simulink model "BoatLibraryTest02"  (R2013b)
settings: Solver=ode45  StartTime=0.0  StopTime=10  RelTol=1e-3
values from neighbouring files (symbols this model uses):
  C = C0    [Minimizer.m]    (also in parameters2.m = [1 0 0 0 0 0;0 0 1 0 0 0;0 0 0 0 1 0]; parameters3.m = [1 0 0 0 0 0;0 0 1 0 0 0;0 0 0 0 1 0])
  fw = 4    [parameters2.m]    (also in parameters3.m)
  I = 1/12*M*((2*rx1)^2 + (2*ry1)^2)    (= 7.46230507536)    [BoatController.m]    (also in boatDynamics.m; parameters2.m = 20; parameters3.m)
  inputBound = [minInput maxInput]    [parameters3.m]
  kr = 2    [parameters2.m]    (also in parameters3.m)
  M = 80*lbtokg    (= 36.28736)    [BoatController.m]    (also in parameters2.m = 10; parameters3.m)
  rx1 = -12*intom    (= -0.3048)    [BoatController.m]    (also in boatDynamics.m; costfunction.m; parameters3.m)
  rx2 = 12*intom    (= 0.3048)    [BoatController.m]    (also in boatDynamics.m; costfunction.m; parameters3.m)
  ry1 = -69*intom/2 + 6*intom    (= -0.7239)    [BoatController.m]    (also in boatDynamics.m; costfunction.m; parameters3.m)
  ry2 = ry1    (= -0.7239)    [BoatController.m]    (also in boatDynamics.m; costfunction.m; parameters3.m)
undefined symbols (not defined in the file): K
libraries: simulink x6
settings Model: Creator=Darsan  LastModifiedBy=darsan13
settings DataIOCC: SignalLoggingSaveFormat=ModelDataLogs
settings OptimizationCC: ExpressionDepthLimit=2147483647
settings DebuggingCC: FcnCallInpInsideContextMsg=EnableAllAsWarning  StateNameClashWarn=warning

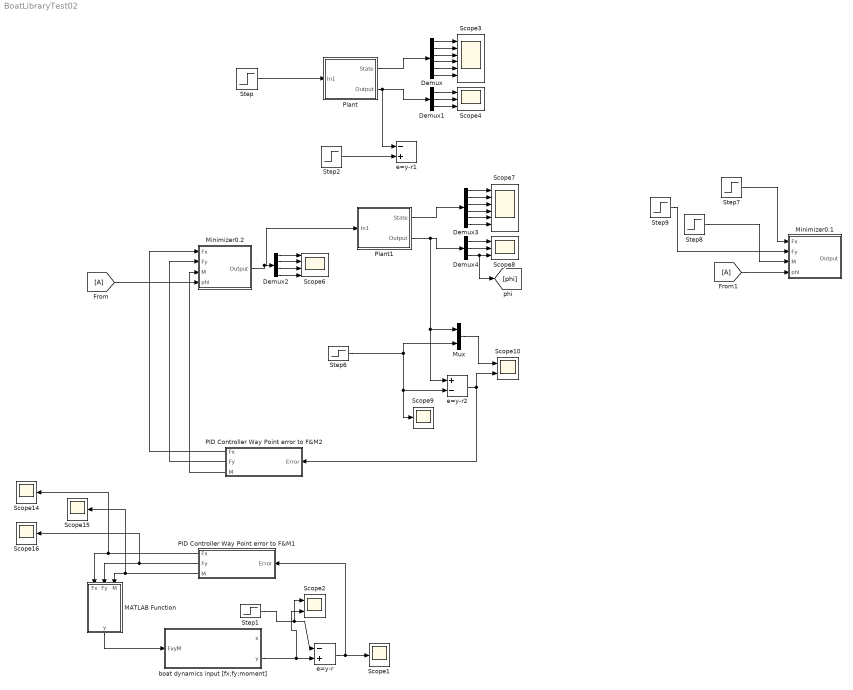
== system BoatLibraryTest02 ==
  Demux : Demux  Outputs=6
  Demux1 : Demux  Outputs=3
  Demux2 : Demux
  Demux3 : Demux  Outputs=6
  Demux4 : Demux  Outputs=3
  MATLAB Function : MATLAB Function  TreatAsAtomicUnit=on
  Minimizer0.1 : Subsystem  mask{rx1=rx1, rx2=rx2, ry1=ry1, ry2=ry2, C=K, inputBound=inputBound}
      mask prompts: C "Performance Gain"; inputBound "Input Bounds"
  Minimizer0.2 : Subsystem  mask{rx1=rx1, rx2=rx2, ry1=ry1, ry2=ry2, C=K, inputBound=inputBound}
      mask prompts: C "Performance Gain"; inputBound "Input Bounds"
  Mux : Mux  Inputs=2
  PID Controller Way Point error to F&M1 : Subsystem
  PID Controller Way Point error to F&M2 : Subsystem
  Plant : Subsystem  mask{rx1=rx1, rx2=rx2, ry1=ry1, ry2=ry2, M=M, I=I, C=C}
      mask TypeOptions rx1: Constant/Value
  Plant1 : Subsystem  mask{rx1=rx1, rx2=rx2, ry1=ry1, ry2=ry2, M=M, I=I, C=C}
      mask TypeOptions rx1: Constant/Value
  Scope{1,9,14..16} (5 alike) : Scope
      Scope1 settings: YMin=-3  YMax=0  SaveName=ScopeData2
      Scope14 settings: YMin=50  YMax=260  SaveName=ScopeData13
      Scope15 settings: YMin=50  YMax=260  SaveName=ScopeData14
      Scope16 settings: YMin=50  YMax=260  SaveName=ScopeData15
      Scope9 settings: SaveName=ScopeData8
  Scope10 : Scope  NumInputPorts=2
      settings: YMin=-22.5~-22.5  YMax=7.5~5  SaveName=ScopeData9
  Scope2 : Scope  NumInputPorts=2
      settings: YMin=-5~-5  YMax=5~5
  Scope3 : Scope  NumInputPorts=6
      settings: YMin=-250000~-4.5~-5~-5~-5~-5  YMax=250000~4.5~5~5~5~5
  Scope4 : Scope  NumInputPorts=3
      settings: YMin=-250000~-4.5~-5  YMax=250000~4.5~5  SaveName=ScopeData3
  Scope6 : Scope  NumInputPorts=4
      settings: YMin=100~100~50~55  YMax=100~100~50~100  SaveName=ScopeData5
  Scope7 : Scope  NumInputPorts=6
      settings: YMin=-250000~-4.5~-5~-5~-5~-5  YMax=250000~4.5~5~5~5~5  SaveName=ScopeData6
  Scope8 : Scope  NumInputPorts=3
      settings: YMin=-220~-440~-1550  YMax=-145~-290~-850  SaveName=ScopeData7
  Step : Step  Before=[0;0;0;0]  After=[-50;.7856;-100;.2961]  SampleTime=0
  Step1 : Step  Before=[0;0;0]  After=[0;1;10]  SampleTime=0
  Step2 : Step  Before=[0;0;0]  After=[0;200;90]  SampleTime=0
  Step6 : Step  Before=[0;0;0]  After=[1;0;0]  SampleTime=0
  Step7 : Step  After=0  SampleTime=0
  Step8 : Step  After=0  SampleTime=0
  Step9 : Step  SampleTime=0
  boat dynamics input [fx;fy;moment] : Subsystem  mask{M=M, I=I, fw=fw, kr=kr, C=C}
      mask prompts: M "Mass"; I "Inert"; fw "Water Friction"; kr "Rotational water Friction"; C "Output Matrix"
  e=y-r : Sum  Inputs=-+
  e=y-r1 : Sum  Inputs=-+
  e=y-r2 : Sum  Inputs=+-
  wires:
  Step1/1 -> Scope2/1, e=y-r/1
  e=y-r/1 -> PID Controller Way Point error to F&M1/1(Error), Scope1/1
  Demux/1 -> Scope3/1
  Demux/2 -> Scope3/2
  Demux/3 -> Scope3/3
  Demux/4 -> Scope3/4
  Demux/5 -> Scope3/5
  Demux/6 -> Scope3/6
  Plant/1(State) -> Demux/1
  Plant/2(Output) -> Demux1/1, e=y-r1/1
  Demux1/1 -> Scope4/1
  Demux1/2 -> Scope4/2
  Demux1/3 -> Scope4/3
  Step2/1 -> e=y-r1/2
  Demux2/1 -> Scope6/1
  Demux2/2 -> Scope6/2
  Demux2/3 -> Scope6/3
  Demux2/4 -> Scope6/4
  Minimizer0.2/1(Output) -> Demux2/1, Plant1/1(In1)
  Demux3/1 -> Scope7/1
  Demux3/2 -> Scope7/2
  Demux3/3 -> Scope7/3
  Demux3/4 -> Scope7/4
  Demux3/5 -> Scope7/5
  Demux3/6 -> Scope7/6
  Plant1/1(State) -> Demux3/1
  Plant1/2(Output) -> Mux/1, e=y-r2/1, Demux4/1
  Demux4/1 -> Scope8/1
  Demux4/2 -> Scope8/2
  Demux4/3 -> [phi], Scope8/3
  PID Controller Way Point error to F&M1/1(Fx) -> Scope14/1, MATLAB Function/1(Fx)
  MATLAB Function/1(y) -> boat dynamics input [fx;fy;moment]/1(FxyM)
  PID Controller Way Point error to F&M1/2(Fy) -> MATLAB Function/2(Fy), Scope16/1
  PID Controller Way Point error to F&M1/3(M) -> Scope15/1, MATLAB Function/3(M)
  Step/1 -> Plant/1(In1)
  boat dynamics input [fx;fy;moment]/2(y) -> Scope2/2, e=y-r/2
  Step6/1 -> e=y-r2/2, Scope9/1, Mux/2
  e=y-r2/1 -> PID Controller Way Point error to F&M2/1(Error), Scope10/2
  [A] -> Minimizer0.2/4(phi)
  Mux/1 -> Scope10/1
  [A] -> Minimizer0.1/4(phi)
  Step8/1 -> Minimizer0.1/3(M)
  Step9/1 -> Minimizer0.1/2(Fy)
  Step7/1 -> Minimizer0.1/1(Fx)
  PID Controller Way Point error to F&M2/1(Fx) -> Minimizer0.2/1(Fx)
  PID Controller Way Point error to F&M2/2(Fy) -> Minimizer0.2/2(Fy)
  PID Controller Way Point error to F&M2/3(M) -> Minimizer0.2/3(M)

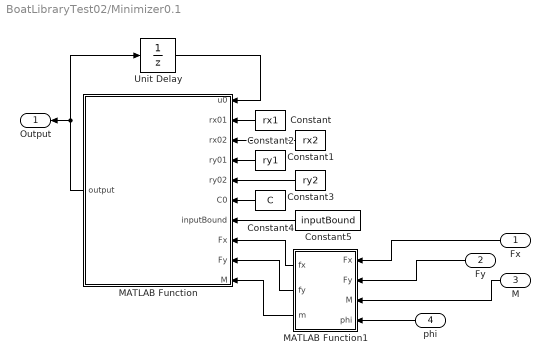
== system BoatLibraryTest02/Minimizer0.1 ==
  Fx : Inport
  Fy : Inport  Port=2
  M : Inport  Port=3
  phi : Inport  Port=4
  Constant : Constant  Value=rx1
  Constant1 : Constant  Value=rx2
  Constant2 : Constant  Value=ry1
  Constant3 : Constant  Value=ry2
  Constant4 : Constant  Value=C
  Constant5 : Constant  Value=inputBound
  MATLAB Function : MATLAB Function  TreatAsAtomicUnit=on
  MATLAB Function1 : MATLAB Function  TreatAsAtomicUnit=on
  Unit Delay : UnitDelay  InitialCondition=[0;0;0;0]  SampleTime=-1
  Output : Outport
  wires:
  Constant/1 -> MATLAB Function/2(rx01)
  Constant1/1 -> MATLAB Function/3(rx02)
  Constant2/1 -> MATLAB Function/4(ry01)
  Constant4/1 -> MATLAB Function/6(C0)
  Unit Delay/1 -> MATLAB Function/1(u0)
  MATLAB Function/1(output) -> Unit Delay/1, Output/1
  Constant5/1 -> MATLAB Function/7(inputBound)
  Constant3/1 -> MATLAB Function/5(ry02)
  MATLAB Function1/3(m) -> MATLAB Function/10(M)
  MATLAB Function1/2(fy) -> MATLAB Function/9(Fy)
  MATLAB Function1/1(fx) -> MATLAB Function/8(Fx)
  Fy/1 -> MATLAB Function1/2(Fy)
  Fx/1 -> MATLAB Function1/1(Fx)
  M/1 -> MATLAB Function1/3(M)
  phi/1 -> MATLAB Function1/4(phi)

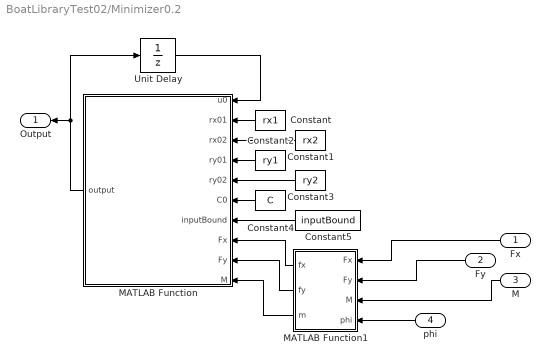
== system BoatLibraryTest02/Minimizer0.2 ==
  Fx : Inport
  Fy : Inport  Port=2
  M : Inport  Port=3
  phi : Inport  Port=4
  Constant : Constant  Value=rx1
  Constant1 : Constant  Value=rx2
  Constant2 : Constant  Value=ry1
  Constant3 : Constant  Value=ry2
  Constant4 : Constant  Value=C
  Constant5 : Constant  Value=inputBound
  MATLAB Function : MATLAB Function  TreatAsAtomicUnit=on
  MATLAB Function1 : MATLAB Function  TreatAsAtomicUnit=on
  Unit Delay : UnitDelay  InitialCondition=[0;0;0;0]  SampleTime=-1
  Output : Outport
  wires:
  Constant/1 -> MATLAB Function/2(rx01)
  Constant1/1 -> MATLAB Function/3(rx02)
  Constant2/1 -> MATLAB Function/4(ry01)
  Constant4/1 -> MATLAB Function/6(C0)
  Unit Delay/1 -> MATLAB Function/1(u0)
  MATLAB Function/1(output) -> Unit Delay/1, Output/1
  Constant5/1 -> MATLAB Function/7(inputBound)
  Constant3/1 -> MATLAB Function/5(ry02)
  MATLAB Function1/3(m) -> MATLAB Function/10(M)
  MATLAB Function1/2(fy) -> MATLAB Function/9(Fy)
  MATLAB Function1/1(fx) -> MATLAB Function/8(Fx)
  Fy/1 -> MATLAB Function1/2(Fy)
  Fx/1 -> MATLAB Function1/1(Fx)
  M/1 -> MATLAB Function1/3(M)
  phi/1 -> MATLAB Function1/4(phi)

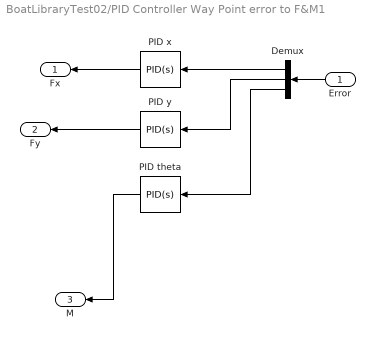
== system BoatLibraryTest02/PID Controller Way Point error to F&M1 ==
  Error : Inport
  Demux : Demux  Outputs=3
  PID theta : simulink/Continuous/PID Controller  Controller=PID  TimeDomain=Continuous-time  SampleTime=1  IntegratorMethod=Forward Euler  FilterMethod=Forward Euler  Form=Parallel  P=-0.684430425608781  I=-0.00538130354417155  D=-7.90308790680083  N=2.12291335792304  InitialConditionSource=internal  InitialConditionForIntegrator=0  InitialConditionForFilter=0  ExternalReset=none  LimitOutput=off  UpperSaturationLimit=inf  LowerSaturationLimit=-inf  LinearizeAsGain=off  AntiWindupMode=none  Kb=1  TrackingMode=off  Kt=1  PParamMin=[]  PParamMax=[]  IParamMin=[]  IParamMax=[]  DParamMin=[]  DParamMax=[]  NParamMin=[]  NParamMax=[]  KbParamMin=[]  KbParamMax=[]  KtParamMin=[]  KtParamMax=[]  POutMin=[]  POutMax=[]  IOutMin=[]  IOutMax=[]  DOutMin=[]  DOutMax=[]  NOutMin=[]  NOutMax=[]  KbOutMin=[]  KbOutMax=[]  KtOutMin=[]  KtOutMax=[]  IntegratorOutMin=[]  IntegratorOutMax=[]  FilterOutMin=[]  FilterOutMax=[]  SumOutMin=[]  SumOutMax=[]  SumI1OutMin=[]  SumI1OutMax=[]  SumI2OutMin=[]  SumI2OutMax=[]  SumI3OutMin=[]  SumI3OutMax=[]  SumDOutMin=[]  SumDOutMax=[]  SaturationOutMin=[]  SaturationOutMax=[]  IntegratorContinuousStateAttributes=''  IntegratorStateMustResolveToSignalObject=off  IntegratorRTWStateStorageClass=Auto  FilterContinuousStateAttributes=''  FilterStateMustResolveToSignalObject=off  FilterRTWStateStorageClass=Auto
  PID x : simulink/Continuous/PID Controller  Controller=PID  TimeDomain=Continuous-time  SampleTime=1  IntegratorMethod=Forward Euler  FilterMethod=Forward Euler  Form=Parallel  P=-3.3282173535127  I=-0.0261679597664008  D=-38.4307788397264  N=2.12291335792304  InitialConditionSource=internal  InitialConditionForIntegrator=0  InitialConditionForFilter=0  ExternalReset=none  LimitOutput=off  UpperSaturationLimit=inf  LowerSaturationLimit=-inf  LinearizeAsGain=off  AntiWindupMode=none  Kb=1  TrackingMode=off  Kt=1  PParamMin=[]  PParamMax=[]  IParamMin=[]  IParamMax=[]  DParamMin=[]  DParamMax=[]  NParamMin=[]  NParamMax=[]  KbParamMin=[]  KbParamMax=[]  KtParamMin=[]  KtParamMax=[]  POutMin=[]  POutMax=[]  IOutMin=[]  IOutMax=[]  DOutMin=[]  DOutMax=[]  NOutMin=[]  NOutMax=[]  KbOutMin=[]  KbOutMax=[]  KtOutMin=[]  KtOutMax=[]  IntegratorOutMin=[]  IntegratorOutMax=[]  FilterOutMin=[]  FilterOutMax=[]  SumOutMin=[]  SumOutMax=[]  SumI1OutMin=[]  SumI1OutMax=[]  SumI2OutMin=[]  SumI2OutMax=[]  SumI3OutMin=[]  SumI3OutMax=[]  SumDOutMin=[]  SumDOutMax=[]  SaturationOutMin=[]  SaturationOutMax=[]  IntegratorContinuousStateAttributes=''  IntegratorStateMustResolveToSignalObject=off  IntegratorRTWStateStorageClass=Auto  FilterContinuousStateAttributes=''  FilterStateMustResolveToSignalObject=off  FilterRTWStateStorageClass=Auto
  PID y : simulink/Continuous/PID Controller  Controller=PID  TimeDomain=Continuous-time  SampleTime=1  IntegratorMethod=Forward Euler  FilterMethod=Forward Euler  Form=Parallel  P=-3.3282173535127  I=-0.0261679597664008  D=-38.4307788397264  N=2.12291335792304  InitialConditionSource=internal  InitialConditionForIntegrator=0  InitialConditionForFilter=0  ExternalReset=none  LimitOutput=off  UpperSaturationLimit=inf  LowerSaturationLimit=-inf  LinearizeAsGain=off  AntiWindupMode=none  Kb=1  TrackingMode=off  Kt=1  PParamMin=[]  PParamMax=[]  IParamMin=[]  IParamMax=[]  DParamMin=[]  DParamMax=[]  NParamMin=[]  NParamMax=[]  KbParamMin=[]  KbParamMax=[]  KtParamMin=[]  KtParamMax=[]  POutMin=[]  POutMax=[]  IOutMin=[]  IOutMax=[]  DOutMin=[]  DOutMax=[]  NOutMin=[]  NOutMax=[]  KbOutMin=[]  KbOutMax=[]  KtOutMin=[]  KtOutMax=[]  IntegratorOutMin=[]  IntegratorOutMax=[]  FilterOutMin=[]  FilterOutMax=[]  SumOutMin=[]  SumOutMax=[]  SumI1OutMin=[]  SumI1OutMax=[]  SumI2OutMin=[]  SumI2OutMax=[]  SumI3OutMin=[]  SumI3OutMax=[]  SumDOutMin=[]  SumDOutMax=[]  SaturationOutMin=[]  SaturationOutMax=[]  IntegratorContinuousStateAttributes=''  IntegratorStateMustResolveToSignalObject=off  IntegratorRTWStateStorageClass=Auto  FilterContinuousStateAttributes=''  FilterStateMustResolveToSignalObject=off  FilterRTWStateStorageClass=Auto
  Fx : Outport
  Fy : Outport  Port=2
  M : Outport  Port=3
  wires:
  Demux/1 -> PID x/1
  Demux/2 -> PID y/1
  Demux/3 -> PID theta/1
  Error/1 -> Demux/1
  PID y/1 -> Fy/1
  PID x/1 -> Fx/1
  PID theta/1 -> M/1

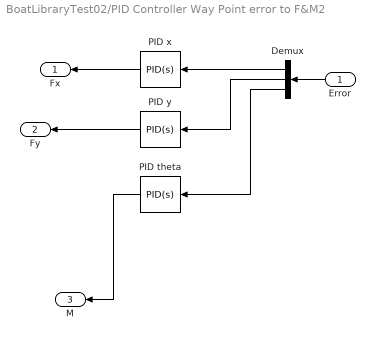
== system BoatLibraryTest02/PID Controller Way Point error to F&M2 ==
  Error : Inport
  Demux : Demux  Outputs=3
  PID theta : simulink/Continuous/PID Controller  Controller=PID  TimeDomain=Continuous-time  SampleTime=1  IntegratorMethod=Forward Euler  FilterMethod=Forward Euler  Form=Parallel  P=-0.684430425608781  I=-0.00538130354417155  D=-7.90308790680083  N=2.12291335792304  InitialConditionSource=internal  InitialConditionForIntegrator=0  InitialConditionForFilter=0  ExternalReset=none  LimitOutput=off  UpperSaturationLimit=inf  LowerSaturationLimit=-inf  LinearizeAsGain=off  AntiWindupMode=none  Kb=1  TrackingMode=off  Kt=1  PParamMin=[]  PParamMax=[]  IParamMin=[]  IParamMax=[]  DParamMin=[]  DParamMax=[]  NParamMin=[]  NParamMax=[]  KbParamMin=[]  KbParamMax=[]  KtParamMin=[]  KtParamMax=[]  POutMin=[]  POutMax=[]  IOutMin=[]  IOutMax=[]  DOutMin=[]  DOutMax=[]  NOutMin=[]  NOutMax=[]  KbOutMin=[]  KbOutMax=[]  KtOutMin=[]  KtOutMax=[]  IntegratorOutMin=[]  IntegratorOutMax=[]  FilterOutMin=[]  FilterOutMax=[]  SumOutMin=[]  SumOutMax=[]  SumI1OutMin=[]  SumI1OutMax=[]  SumI2OutMin=[]  SumI2OutMax=[]  SumI3OutMin=[]  SumI3OutMax=[]  SumDOutMin=[]  SumDOutMax=[]  SaturationOutMin=[]  SaturationOutMax=[]  IntegratorContinuousStateAttributes=''  IntegratorStateMustResolveToSignalObject=off  IntegratorRTWStateStorageClass=Auto  FilterContinuousStateAttributes=''  FilterStateMustResolveToSignalObject=off  FilterRTWStateStorageClass=Auto
  PID x : simulink/Continuous/PID Controller  Controller=PID  TimeDomain=Continuous-time  SampleTime=1  IntegratorMethod=Forward Euler  FilterMethod=Forward Euler  Form=Parallel  P=-3.3282173535127  I=-0.0261679597664008  D=-38.4307788397264  N=2.12291335792304  InitialConditionSource=internal  InitialConditionForIntegrator=0  InitialConditionForFilter=0  ExternalReset=none  LimitOutput=off  UpperSaturationLimit=inf  LowerSaturationLimit=-inf  LinearizeAsGain=off  AntiWindupMode=none  Kb=1  TrackingMode=off  Kt=1  PParamMin=[]  PParamMax=[]  IParamMin=[]  IParamMax=[]  DParamMin=[]  DParamMax=[]  NParamMin=[]  NParamMax=[]  KbParamMin=[]  KbParamMax=[]  KtParamMin=[]  KtParamMax=[]  POutMin=[]  POutMax=[]  IOutMin=[]  IOutMax=[]  DOutMin=[]  DOutMax=[]  NOutMin=[]  NOutMax=[]  KbOutMin=[]  KbOutMax=[]  KtOutMin=[]  KtOutMax=[]  IntegratorOutMin=[]  IntegratorOutMax=[]  FilterOutMin=[]  FilterOutMax=[]  SumOutMin=[]  SumOutMax=[]  SumI1OutMin=[]  SumI1OutMax=[]  SumI2OutMin=[]  SumI2OutMax=[]  SumI3OutMin=[]  SumI3OutMax=[]  SumDOutMin=[]  SumDOutMax=[]  SaturationOutMin=[]  SaturationOutMax=[]  IntegratorContinuousStateAttributes=''  IntegratorStateMustResolveToSignalObject=off  IntegratorRTWStateStorageClass=Auto  FilterContinuousStateAttributes=''  FilterStateMustResolveToSignalObject=off  FilterRTWStateStorageClass=Auto
  PID y : simulink/Continuous/PID Controller  Controller=PID  TimeDomain=Continuous-time  SampleTime=1  IntegratorMethod=Forward Euler  FilterMethod=Forward Euler  Form=Parallel  P=-3.3282173535127  I=-0.0261679597664008  D=-38.4307788397264  N=2.12291335792304  InitialConditionSource=internal  InitialConditionForIntegrator=0  InitialConditionForFilter=0  ExternalReset=none  LimitOutput=off  UpperSaturationLimit=inf  LowerSaturationLimit=-inf  LinearizeAsGain=off  AntiWindupMode=none  Kb=1  TrackingMode=off  Kt=1  PParamMin=[]  PParamMax=[]  IParamMin=[]  IParamMax=[]  DParamMin=[]  DParamMax=[]  NParamMin=[]  NParamMax=[]  KbParamMin=[]  KbParamMax=[]  KtParamMin=[]  KtParamMax=[]  POutMin=[]  POutMax=[]  IOutMin=[]  IOutMax=[]  DOutMin=[]  DOutMax=[]  NOutMin=[]  NOutMax=[]  KbOutMin=[]  KbOutMax=[]  KtOutMin=[]  KtOutMax=[]  IntegratorOutMin=[]  IntegratorOutMax=[]  FilterOutMin=[]  FilterOutMax=[]  SumOutMin=[]  SumOutMax=[]  SumI1OutMin=[]  SumI1OutMax=[]  SumI2OutMin=[]  SumI2OutMax=[]  SumI3OutMin=[]  SumI3OutMax=[]  SumDOutMin=[]  SumDOutMax=[]  SaturationOutMin=[]  SaturationOutMax=[]  IntegratorContinuousStateAttributes=''  IntegratorStateMustResolveToSignalObject=off  IntegratorRTWStateStorageClass=Auto  FilterContinuousStateAttributes=''  FilterStateMustResolveToSignalObject=off  FilterRTWStateStorageClass=Auto
  Fx : Outport
  Fy : Outport  Port=2
  M : Outport  Port=3
  wires:
  Demux/1 -> PID x/1
  Demux/2 -> PID y/1
  Demux/3 -> PID theta/1
  Error/1 -> Demux/1
  PID y/1 -> Fy/1
  PID x/1 -> Fx/1
  PID theta/1 -> M/1

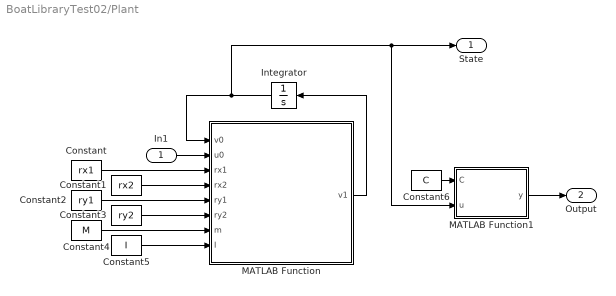
== system BoatLibraryTest02/Plant ==
  In1 : Inport
  Constant : Constant  Value=rx1
  Constant1 : Constant  Value=rx2
  Constant2 : Constant  Value=ry1
  Constant3 : Constant  Value=ry2
  Constant4 : Constant  Value=M
  Constant5 : Constant  Value=I
  Constant6 : Constant  Value=C
  Integrator : Integrator  InitialCondition=[0 0 0 0 0 0]
  MATLAB Function : MATLAB Function  TreatAsAtomicUnit=on
  MATLAB Function1 : MATLAB Function  TreatAsAtomicUnit=on
  State : Outport
  Output : Outport  Port=2
  wires:
  Constant/1 -> MATLAB Function/3(rx1)
  Constant1/1 -> MATLAB Function/4(rx2)
  Constant2/1 -> MATLAB Function/5(ry1)
  Constant3/1 -> MATLAB Function/6(ry2)
  Constant4/1 -> MATLAB Function/7(m)
  Constant5/1 -> MATLAB Function/8(I)
  MATLAB Function/1(v1) -> Integrator/1
  Integrator/1 -> MATLAB Function/1(v0), State/1, MATLAB Function1/2(u)
  In1/1 -> MATLAB Function/2(u0)
  Constant6/1 -> MATLAB Function1/1(C)
  MATLAB Function1/1(y) -> Output/1

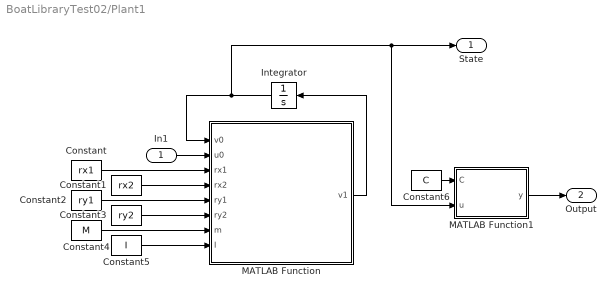
== system BoatLibraryTest02/Plant1 ==
  In1 : Inport
  Constant : Constant  Value=rx1
  Constant1 : Constant  Value=rx2
  Constant2 : Constant  Value=ry1
  Constant3 : Constant  Value=ry2
  Constant4 : Constant  Value=M
  Constant5 : Constant  Value=I
  Constant6 : Constant  Value=C
  Integrator : Integrator  InitialCondition=[0 0 0 0 0 0]
  MATLAB Function : MATLAB Function  TreatAsAtomicUnit=on
  MATLAB Function1 : MATLAB Function  TreatAsAtomicUnit=on
  State : Outport
  Output : Outport  Port=2
  wires:
  Constant/1 -> MATLAB Function/3(rx1)
  Constant1/1 -> MATLAB Function/4(rx2)
  Constant2/1 -> MATLAB Function/5(ry1)
  Constant3/1 -> MATLAB Function/6(ry2)
  Constant4/1 -> MATLAB Function/7(m)
  Constant5/1 -> MATLAB Function/8(I)
  MATLAB Function/1(v1) -> Integrator/1
  Integrator/1 -> MATLAB Function/1(v0), State/1, MATLAB Function1/2(u)
  In1/1 -> MATLAB Function/2(u0)
  Constant6/1 -> MATLAB Function1/1(C)
  MATLAB Function1/1(y) -> Output/1

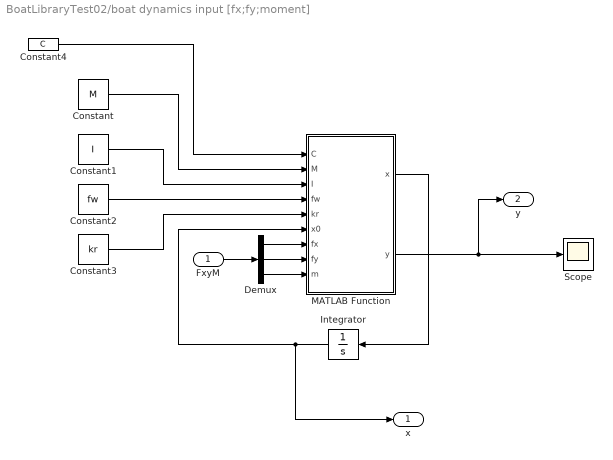
== system BoatLibraryTest02/boat dynamics input [fx;fy;moment] ==
  FxyM : Inport
  Constant : Constant  Value=M
  Constant1 : Constant  Value=I
  Constant2 : Constant  Value=fw
  Constant3 : Constant  Value=kr
  Constant4 : Constant  Value=C
  Demux : Demux  Outputs=3
  Integrator : Integrator  InitialCondition=[0 0 0 0 0 0]
  MATLAB Function : MATLAB Function  TreatAsAtomicUnit=on
  Scope : Scope
  x : Outport
  y : Outport  Port=2
  wires:
  MATLAB Function/2(y) -> Scope/1, y/1
  Integrator/1 -> x/1, MATLAB Function/6(x0)
  Constant/1 -> MATLAB Function/2(M)
  Constant1/1 -> MATLAB Function/3(I)
  Constant2/1 -> MATLAB Function/4(fw)
  Constant3/1 -> MATLAB Function/5(kr)
  Constant4/1 -> MATLAB Function/1(C)
  MATLAB Function/1(x) -> Integrator/1
  FxyM/1 -> Demux/1
  Demux/1 -> MATLAB Function/7(fx)
  Demux/2 -> MATLAB Function/8(fy)
  Demux/3 -> MATLAB Function/9(m)

== matlab function BoatLibraryTest02/Plant/MATLAB Function ==
  data: v0 input; v1 output; u0 input; rx1 input; rx2 input; ry1 input; ry2 input; m input; I input
function v1   = boatDynamics(v0, u0, rx1, rx2, ry1, ry2, m, I)

    % %%%%%%%%%%%%%%%%%%%%%%%%%%%%%%%%%%%%%%%%%%%% %
    %    v = [x...          %    u = [theta1...    %
    %        x_dot...       %        f1...         %
    %        y...           %        theta2...     %
    %        y_dot...       %        f2]           %
    %        theta...       %                      %
    %        theta_dot];    %                      %
    % %%%%%%%%%%%%%%%%%%%%%%%%%%%%%%%%%%%%%%%%%%%% %
    
    v11 = v0(2);
    v12 = -u0(2)/m*sind(u0(1)+v0(5)) - u0(4)/m*sind(u0(3)+v0(5)) - 0*5*v0(1);
    v13 = v0(4);
    v14 = u0(2)/m*cosd(u0(1)+v0(5)) + u0(4)/m*cosd(u0(3)+v0(5)) - 0*2*v0(3);
    v15 = v0(6);
    v16 = rx1/I*u0(2)*cosd(u0(1)) + ry1/I*u0(2)*sind(u0(1)) + rx2/I*u0(4)*cosd(u0(3)) + ry2/I*u0(4)*sind(u0(3)) - 0*9*v0(5);
   
    v1 = [v11;v12;v13;v14;v15;v16];
    
    
end

== matlab function BoatLibraryTest02/boat dynamics input [fx;fy;moment]/MATLAB Function ==
  data: C input; x output; M input; I input; fw input; kr input; x0 input; fx input; y output; fy input; m input
function [x,y] = systemstep(C,M,I,fw,kr,x0,fx,fy,m)

   % status vector y=[x;x_dot;y;_y_dot;theta;theta_dot]
   % forces u=[fx;fy;m]
   % contant parameters {mass; rotational inertia; friction coefficients }
   
   x1 = x0(2);
   x2 = fx/M - x0(2)*fw*0;
   x3 = x0(4);
   x4 = fy/M - x0(4)*fw*0;
   x5 = x0(6);
   x6 = m/I - x0(6)*kr*0;

   x=[x1;x2;x3;x4;x5;x6];
   
   y = C*x0;

== matlab function BoatLibraryTest02/Plant/MATLAB Function1 ==
  data: C input; u input; y output
function y = fcn(C,u)
%#codegen

y = C*u;

== matlab function BoatLibraryTest02/Plant1/MATLAB Function ==
  data: v0 input; v1 output; u0 input; rx1 input; rx2 input; ry1 input; ry2 input; m input; I input
function v1   = boatDynamics(v0, u0, rx1, rx2, ry1, ry2, m, I)

    % %%%%%%%%%%%%%%%%%%%%%%%%%%%%%%%%%%%%%%%%%%%% %
    %    v = [x...          %    u = [theta1...    %
    %        x_dot...       %        f1...         %
    %        y...           %        theta2...     %
    %        y_dot...       %        f2]           %
    %        theta...       %                      %
    %        theta_dot];    %                      %
    % %%%%%%%%%%%%%%%%%%%%%%%%%%%%%%%%%%%%%%%%%%%% %
    
    v11 = v0(2);
    v12 = -u0(2)/m*sind(u0(1)+v0(5)) - u0(4)/m*sind(u0(3)+v0(5)) - 0*5*v0(1);
    v13 = v0(4);
    v14 = u0(2)/m*cosd(u0(1)+v0(5)) + u0(4)/m*cosd(u0(3)+v0(5)) - 0*2*v0(3);
    v15 = v0(6);
    v16 = rx1/I*u0(2)*cosd(u0(1)) + ry1/I*u0(2)*sind(u0(1)) + rx2/I*u0(4)*cosd(u0(3)) + ry2/I*u0(4)*sind(u0(3)) - 0*9*v0(5);
   
    v1 = [v11;v12;v13;v14;v15;v16];
    
    
end

== matlab function BoatLibraryTest02/Plant1/MATLAB Function1 ==
  data: C input; u input; y output
function y = fcn(C,u)
%#codegen

y = C*u;

== matlab function BoatLibraryTest02/MATLAB Function ==
  data: Fx input; y output; Fy input; M input
function y = fcn(Fx,Fy,M)
%#codegen

y = [Fx;Fy;M];

== matlab function BoatLibraryTest02/Minimizer0.1/MATLAB Function ==
  data: u0 input; output output; rx01 input; rx02 input; ry01 input; ry02 input; C0 input; inputBound input; Fx input; Fy input; M input
function output = Minimizer(u0, rx01, rx02, ry01, ry02, C0, inputBound, Fx, Fy, M)

rx1 = rx01; rx2 = rx02;
ry1 = ry01; ry2 = ry02;

C = C0;

Fxref = Fx; Fyref = Fy; Mref  = M;

gridNum = 5;

grid = boundGrid(inputBound, gridNum);

% u1 = getMinFromGrid(grid, u0, Fxref, Fyref, Mref, rx1, rx2, ry1, ry2, C);

u1 = u0;

    for k = 1:100
        h = getDirection(u1, u0, Fxref, Fyref, Mref, rx1, rx2, ry1, ry2, C);
        alpha = getStepSize(u1, u0, h, Fxref, Fyref, Mref, rx1, rx2, ry1, ry2, C);
        u1 = u1 + alpha*h;
        u1 = checkInputBound(u1,inputBound);
    end
    
    output = u1;

end

function output = getMinFromGrid(grid, preinput, Fxref, Fyref, Mref, rx1, rx2, ry1, ry2, C)

[ii, iii] = size(grid);
v0 = costFunction(grid(1,:), preinput, Fxref, Fyref, Mref, rx1, rx2, ry1, ry2, C);

output = [grid(1,1);grid(1,2);grid(1,3);grid(1,4)];

for i = 1:ii
    for j = 1:ii
        for k = 1:ii
            for l = 1:ii
                input = [grid(i,1);grid(j,2);grid(k,3);grid(l,4)];
                v1 = costFunction(input,preinput, Fxref, Fyref, Mref, rx1, rx2, ry1, ry2, C);
                if v0 > v1
                    v0 = v1;
                    output = input;
                else                 
                end
            end
        end
    end
end

end

function output = checkInputBound(input,inputBound)
k = [0;0;0;0];
    for i = 1:length(input)
        k(i) = sat(input(i),inputBound(i,:));
    end
    output = k;
end

function output = boundGrid(inputBound, gridNum)

p = gridNum;

theta1 =    linspace(inputBound(1,1),inputBound(1,2),p)';
f1 =        linspace(inputBound(2,1),inputBound(2,2),p)';
theta2 =    linspace(inputBound(3,1),inputBound(3,2),p)';
f2 =        linspace(inputBound(4,1),inputBound(4,2),p)';

output = [theta1, f1, theta2, f2];

end

function output = sat(input, bound)

    if input < bound(1)
        output = bound(1);
    elseif input > bound(2)
        output = bound(2);
    else
        output = input;
    end

end

function output = getStepSize(input, preinput, h, Fxref, Fyref, Mref, rx1, rx2, ry1, ry2, C)

 alpha = 1;
    
    u0 = input;
    u1 = input + alpha*h;
    
    v0 = costFunction( u0, preinput, Fxref, Fyref, Mref, rx1, rx2, ry1, ry2, C );
    v1 = costFunction( u1, preinput, Fxref, Fyref, Mref, rx1, rx2, ry1, ry2, C );

    while v1 <= v0 && v1 ~= 0
        alpha = alpha + 1;
        u1 = input + alpha*h;
        v0 = v1;
        v1 = costFunction( u1, preinput, Fxref, Fyref, Mref, rx1, rx2, ry1, ry2, C );
    end
    
    v0 = v1;

    while v1 <= v0 && alpha > 0 && v1 ~= 0
        alpha = alpha - 0.01;
        u1 = input + alpha*h;
        v0 = v1;
        v1 = costFunction( u1, preinput, Fxref, Fyref, Mref, rx1, rx2, ry1, ry2, C );
    end
    
    alpha = alpha + 0.01;

    output = alpha;

end

function output = costFunction(input, preinput, Fxref, Fyref, Mref, rx1, rx2, ry1, ry2, C)

    theta1  = input(1);
    f1      = input(2);
    theta2  = input(3);
    f2      = input(4);
    
    pretheta1   = preinput(1);
    pretheta2   = preinput(3);

    Fx = -f1*sind(theta1) - f2*sind(theta2);
    Fy = f1*cosd(theta1) + f2*cosd(theta2);
    M = rx1*f1*cosd(theta1) + ry1*f1*sind(theta1) + rx2*f2*cosd(theta2)...
        + ry2*f2*sind(theta2);

    output = C(1)*(Fx-Fxref)^2 +...
        C(2)*(Fy-Fyref)^2 +...
        C(3)*(M-Mref)^2  +...
        C(4)*f1^2 +...
        C(5)*f2^2 +...
        C(6)*(theta1 - pretheta1)^2 +...
        C(7)*(theta2 - pretheta2)^2;

end

function output = getDirection(input, preinput, Fxref, Fyref, Mref, rx1, rx2, ry1, ry2, C)

hsd = SteepestDescent(input, preinput, Fxref, Fyref, Mref, rx1, rx2, ry1, ry2, C);

output = zeros(4,1);

    for i = 1:length(hsd)
        output(i) = hsd(i);
    end
end

function output = SteepestDescent(input, preinput, Fxref, Fyref, Mref, rx1, rx2, ry1, ry2, C)

theta1  = input(1);
f1      = input(2);
theta2  = input(3);
f2      = input(4);

pretheta1   = preinput(1);
pretheta2   = preinput(3);

dVdtheta1 = C(3)*(f1*ry1*cosd(theta1)...
    - f1*rx1*sind(theta1))*(f1*rx1*cosd(theta1)...
    - Mref + f2*rx2*cosd(theta2) + f1*ry1*sin(theta1)...
    + f2*ry2*sind(theta2)) - C(6)*(pretheta1 - theta1)...
    - C(2)*f1*sind(theta1)*(f1*cosd(theta1) - Fyref + f2*cosd(theta2))...
    + C(1)*f1*cosd(theta1)*(Fxref + f1*sind(theta1) + f2*sind(theta2));

dVdf1 = C(4)*f1 + C(1)*sind(theta1)*(Fxref + f1*sin(theta1)...
    + f2*sind(theta2)) + C(2)*cosd(theta1)*(f1*cosd(theta1) - Fyref...
    + f2*cosd(theta2)) + C(3)*(rx1*cosd(theta1)...
    + ry1*sind(theta1))*(f1*rx1*cosd(theta1) - Mref + f2*rx2*cosd(theta2)...
    + f1*ry1*sind(theta1) + f2*ry2*sind(theta2));

dVdtheta2 = C(3)*(f2*ry2*cosd(theta2)...
    - f2*rx2*sind(theta2))*(f1*rx1*cosd(theta1)...
    - Mref + f2*rx2*cosd(theta2) + f1*ry1*sind(theta1)...
    + f2*ry2*sind(theta2)) - C(7)*(pretheta2 - theta2)...
    - C(2)*f2*sind(theta2)*(f1*cosd(theta1) - Fyref + f2*cosd(theta2))...
    + C(1)*f2*cosd(theta2)*(Fxref + f1*sind(theta1) + f2*sind(theta2));

dVdf2 = C(5)*f2 + C(1)*sind(theta2)*(Fxref + f1*sind(theta1)...
    + f2*sind(theta2)) + C(2)*cosd(theta2)*(f1*cosd(theta1) - Fyref...
    + f2*cosd(theta2)) + C(3)*(rx2*cosd(theta2)...
    + ry2*sind(theta2))*(f1*rx1*cosd(theta1) - Mref + f2*rx2*cosd(theta2)...
    + f1*ry1*sind(theta1) + f2*ry2*sind(theta2));
 
output = -[dVdtheta1; dVdf1; dVdtheta2; dVdf2];

end

== matlab function BoatLibraryTest02/Minimizer0.1/MATLAB Function1 ==
  data: Fx input; fx output; Fy input; M input; fy output; m output; phi input
function [fx,fy,m] = fcn(Fx,Fy,M, phi)
%#codegen

R = [cosd(phi) -sin(phi) 0;...
        sind(phi)  cos(phi) 0;...
        0           0       1];
    
    FxyM = R*[Fx;Fy;M];
    
    fx = FxyM(1);
    fy = FxyM(2);
    m = FxyM(3);
    
end

== matlab function BoatLibraryTest02/Minimizer0.2/MATLAB Function ==
  data: u0 input; output output; rx01 input; rx02 input; ry01 input; ry02 input; C0 input; inputBound input; Fx input; Fy input; M input
function output = Minimizer(u0, rx01, rx02, ry01, ry02, C0, inputBound, Fx, Fy, M)

rx1 = rx01; rx2 = rx02;
ry1 = ry01; ry2 = ry02;

C = C0;

Fxref = Fx; Fyref = Fy; Mref  = M;

gridNum = 5;

grid = boundGrid(inputBound, gridNum, rx1,ry1);

u1 = getMinFromGrid(grid, u0, Fxref, Fyref, Mref, rx1, rx2, ry1, ry2, C);

% u1 = u0;

    for k = 1:20
        h = getDirection(u1, u0, Fxref, Fyref, Mref, rx1, rx2, ry1, ry2, C);
        alpha = getStepSize(u1, u0, h, Fxref, Fyref, Mref, rx1, rx2, ry1, ry2, C);
        u1 = u1 + alpha*h;
        u1 = checkInputBound(u1,inputBound);
    end
    
    output = u1;

end

function output = getMinFromGrid(grid, preinput, Fxref, Fyref, Mref, rx1, rx2, ry1, ry2, C)

[ii, iii] = size(grid);
v0 = costFunction(grid(1,:), preinput, Fxref, Fyref, Mref, rx1, rx2, ry1, ry2, C);

output = [grid(1,1);grid(1,2);grid(1,3);grid(1,4)];

for i = 1:ii
    for j = 1:ii
        for k = 1:ii
            for l = 1:ii
                input = [grid(i,1);grid(j,2);grid(k,3);grid(l,4)];
                v1 = costFunction(input,preinput, Fxref, Fyref, Mref, rx1, rx2, ry1, ry2, C);
                if v0 > v1
                    v0 = v1;
                    output = input;
                else
                end
            end
        end
    end
end

end

function output = checkInputBound(input,inputBound)
k = [0;0;0;0];
    for i = 1:length(input)
        k(i) = sat(input(i),inputBound(i,:));
    end
    output = k;
end

function output = boundGrid(inputBound, gridNum, rx1,ry1)

p = gridNum;

theta1 =    linspace(inputBound(1,1),inputBound(1,2),p)';
f1 =        linspace(inputBound(2,1),inputBound(2,2),p)';
theta2 =    linspace(inputBound(3,1),inputBound(3,2),p)';
f2 =        linspace(inputBound(4,1),inputBound(4,2),p)';

i = atan(rx1/ry1)*180/pi;

output = [theta1, f1, theta2, f2;...
            0,    1,    0,    1;...
           -i,   -1,   -i,   -1;...
            i,    0,    i,    0];

end

function output = sat(input, bound)

    if input < bound(1)
        output = bound(1);
    elseif input > bound(2)
        output = bound(2);
    else
        output = input;
    end

end

function output = getStepSize(input, preinput, h, Fxref, Fyref, Mref, rx1, rx2, ry1, ry2, C)

    alpha = 1;
    
    u0 = input;
    u1 = input + alpha*h;
    
    v0 = costFunction( u0, preinput, Fxref, Fyref, Mref, rx1, rx2, ry1, ry2, C );
    v1 = costFunction( u1, preinput, Fxref, Fyref, Mref, rx1, rx2, ry1, ry2, C );

    while v1 <= v0 && v1 ~= 0
        alpha = alpha + 1;
        u1 = input + alpha*h;
        v0 = v1;
        v1 = costFunction( u1, preinput, Fxref, Fyref, Mref, rx1, rx2, ry1, ry2, C );
    end
    
    v0 = v1;

    while v1 <= v0 && alpha >= 0 && v1 ~= 0
        alpha = alpha - 0.01;
        u1 = input + alpha*h;
        v0 = v1;
        v1 = costFunction( u1, preinput, Fxref, Fyref, Mref, rx1, rx2, ry1, ry2, C );
    end
    
    alpha = alpha + 0.01;

    output = alpha;

end

function output = costFunction(input, preinput, Fxref, Fyref, Mref, rx1, rx2, ry1, ry2, C)

    theta1  = input(1);
    f1      = input(2);
    theta2  = input(3);
    f2      = input(4);
    
    pretheta1   = preinput(1);
    pretheta2   = preinput(3);

    Fx = -f1*sind(theta1) - f2*sind(theta2);
    Fy = f1*cosd(theta1) + f2*cosd(theta2);
    M = rx1*f1*cosd(theta1) + ry1*f1*sind(theta1) + rx2*f2*cosd(theta2)...
        + ry2*f2*sind(theta2);

    output = C(1)*(Fx-Fxref)^2 +...
        C(2)*(Fy-Fyref)^2 +...
        C(3)*(M-Mref)^2  +...
        C(4)*f1^2 +...
        C(5)*f2^2 +...
        C(6)*(theta1 - pretheta1)^2 +...
        C(7)*(theta2 - pretheta2)^2;

end

function output = getDirection(input, preinput, Fxref, Fyref, Mref, rx1, rx2, ry1, ry2, C)

hsd = SteepestDescent(input, preinput, Fxref, Fyref, Mref, rx1, rx2, ry1, ry2, C);

output = zeros(4,1);

    for i = 1:length(hsd)
        output(i) = hsd(i);
    end
    
end

function output = SteepestDescent(input, preinput, Fxref, Fyref, Mref, rx1, rx2, ry1, ry2, C)

theta1  = input(1);
f1      = input(2);
theta2  = input(3);
f2      = input(4);

pretheta1   = preinput(1);
pretheta2   = preinput(3);

dVdtheta1 = C(3)*(f1*ry1*cosd(theta1)...
    - f1*rx1*sind(theta1))*(f1*rx1*cosd(theta1)...
    - Mref + f2*rx2*cosd(theta2) + f1*ry1*sin(theta1)...
    + f2*ry2*sind(theta2)) - C(6)*(pretheta1 - theta1)...
    - C(2)*f1*sind(theta1)*(f1*cosd(theta1) - Fyref + f2*cosd(theta2))...
    + C(1)*f1*cosd(theta1)*(Fxref + f1*sind(theta1) + f2*sind(theta2));

dVdf1 = C(4)*f1 + C(1)*sind(theta1)*(Fxref + f1*sin(theta1)...
    + f2*sind(theta2)) + C(2)*cosd(theta1)*(f1*cosd(theta1) - Fyref...
    + f2*cosd(theta2)) + C(3)*(rx1*cosd(theta1)...
    + ry1*sind(theta1))*(f1*rx1*cosd(theta1) - Mref + f2*rx2*cosd(theta2)...
    + f1*ry1*sind(theta1) + f2*ry2*sind(theta2));

dVdtheta2 = C(3)*(f2*ry2*cosd(theta2)...
    - f2*rx2*sind(theta2))*(f1*rx1*cosd(theta1)...
    - Mref + f2*rx2*cosd(theta2) + f1*ry1*sind(theta1)...
    + f2*ry2*sind(theta2)) - C(7)*(pretheta2 - theta2)...
    - C(2)*f2*sind(theta2)*(f1*cosd(theta1) - Fyref + f2*cosd(theta2))...
    + C(1)*f2*cosd(theta2)*(Fxref + f1*sind(theta1) + f2*sind(theta2));

dVdf2 = C(5)*f2 + C(1)*sind(theta2)*(Fxref + f1*sind(theta1)...
    + f2*sind(theta2)) + C(2)*cosd(theta2)*(f1*cosd(theta1) - Fyref...
    + f2*cosd(theta2)) + C(3)*(rx2*cosd(theta2)...
    + ry2*sind(theta2))*(f1*rx1*cosd(theta1) - Mref + f2*rx2*cosd(theta2)...
    + f1*ry1*sind(theta1) + f2*ry2*sind(theta2));
 
output = -[dVdtheta1; dVdf1; dVdtheta2; dVdf2];

end

== matlab function BoatLibraryTest02/Minimizer0.2/MATLAB Function1 ==
  data: Fx input; fx output; Fy input; M input; fy output; m output; phi input
function [fx,fy,m] = fcn(Fx,Fy,M, phi)
%#codegen

R = [cosd(phi) -sin(phi) 0;...
        sind(phi)  cos(phi) 0;...
        0           0       1];
    
    FxyM = R*[Fx;Fy;M];
    
    fx = FxyM(1);
    fy = FxyM(2);
    m = FxyM(3);
    
end
